simulink model "dinamica_veiculo"  (R2023a)
settings: Solver=VariableStepAuto  StartTime=0.0  StopTime=10.0  RelTol=1e-3
model workspace (MAT data in the model file):
  b = 50
  m = 1000
settings Model: Creator=Alexandre  LastModifiedBy=Alexandre

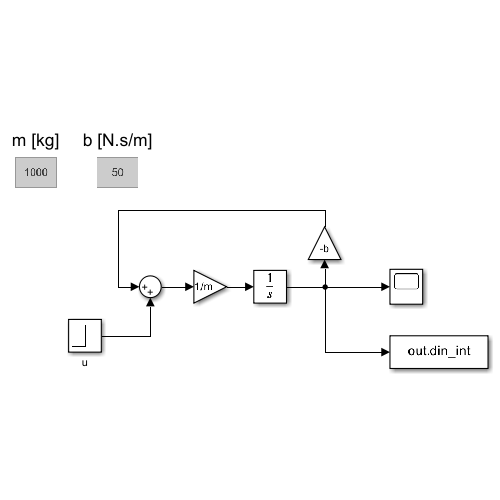
[thumbnail: Simulink's stored preview of the top-level diagram]
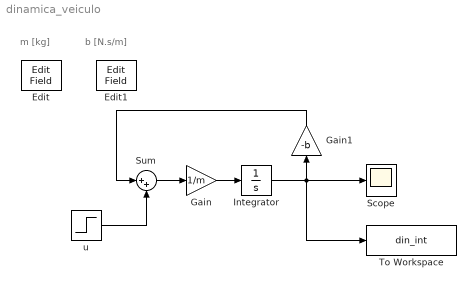
== system dinamica_veiculo ==
  note: m [kg]
  note: b [N.s/m]
  Edit : EditField  LabelPosition=Hide  ShowInitialText=on  Alignment=Center
  Edit1 : EditField  LabelPosition=Hide  ShowInitialText=on  Alignment=Center
  Gain : Gain  Gain=1/m
  Gain1 : Gain  Gain=-b
  Integrator : Integrator
  Scope : Scope
  Sum : Sum  Inputs=|++
  To Workspace : ToWorkspace  VariableName=din_int  SaveFormat=Timeseries  SampleTime=-1
  u : Step  Time=0  After=500  SampleTime=0
  wires:
  u/1 -> Sum/2
  Sum/1 -> Gain/1
  Gain/1 -> Integrator/1
  Integrator/1 -> To Workspace/1, Scope/1, Gain1/1
  Gain1/1 -> Sum/1
